simulink model "perfusion"  (Simulink 8.7)
settings: Solver=ode45  StartTime=0.0  StopTime=24  MaxStep=10  RelTol=1e-3
libraries: simulink x3
settings Model: Creator=asuri  LastModifiedBy=chnam  ExtModeAutoUpdateStatusClock=off
settings SolverCC: ZeroCrossControl=EnableAll
settings DataIOCC: SignalLoggingSaveFormat=ModelDataLogs  SaveOutput=off  SaveTime=off
settings OptimizationCC: BooleanDataType=off  ExpressionDepthLimit=2147483647  InitFltsAndDblsToZero=on
settings DebuggingCC: AlgebraicLoopMsg=error  SaveWithParameterizedLinksMsg=none  SignalResolutionControl=TryResolveAllWithWarning  MultiTaskDSMMsg=warning  MultiTaskCondExecSysMsg=none  InvalidFcnCallConnMsg=warning  FcnCallInpInsideContextMsg=UseLocalSettings  StateNameClashWarn=warning  StrictBusMsg=None
settings SFSimCC: SimParseCustomCode=off
settings GRTTargetCC: TargetFcnLib=ansi_tfl_tmw.mat  GeneratePreprocessorConditionals=Use local settings  CombineOutputUpdateFcns=off  GRTInterface=on

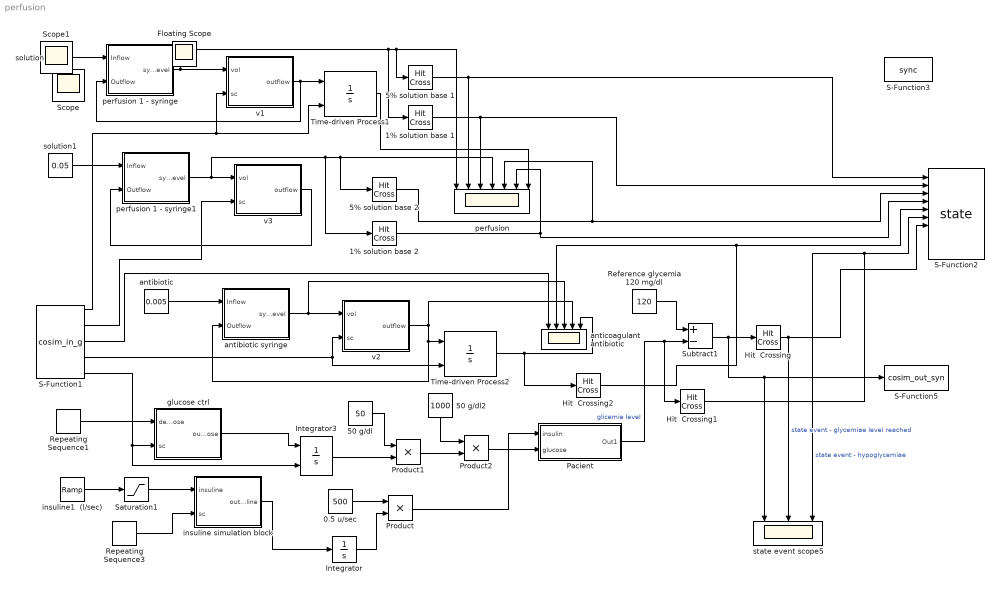
== system perfusion ==
  "0.5 u/sec " : Constant  Value=500
  1% solution base 1 : HitCross  HitCrossingOffset=0.075  HitCrossingDirection=falling  ZeroCross=off
  1% solution base 2 : HitCross  HitCrossingOffset=0.075  HitCrossingDirection=falling  ZeroCross=off
  5% solution base 1 : HitCross  HitCrossingOffset=0.1  HitCrossingDirection=falling  ZeroCross=off
  5% solution base 2 : HitCross  HitCrossingOffset=0.1  HitCrossingDirection=falling  ZeroCross=off
  50 g/dl : Constant  Value=50
  50 g/dl2 : Constant  Value=1000
  Hit  Crossing : HitCross
  Hit  Crossing1 : HitCross  HitCrossingOffset=60  HitCrossingDirection=falling  ZeroCross=off
  Hit  Crossing2 : HitCross  HitCrossingOffset=0.2  HitCrossingDirection=rising  ZeroCross=off
  Integrator : Integrator
  Integrator3 : Integrator  ExternalReset=either
  Pacient : Subsystem
  Product : Product  RndMeth=Zero
  Product1 : Product  RndMeth=Zero
  Product2 : Product  RndMeth=Zero
  "Reference glycemia 120 mg/dl " : Constant  Value=120
  Repeating Sequence1 : simulink/Sources/Repeating Sequence  rep_seq_t=[0 1]  rep_seq_y=[0 0.001]
  Repeating Sequence3 : simulink/Sources/Repeating Sequence  rep_seq_t=[0 1 2 3 4 5 6 7 8 9 10 11 12 13 14 15 16 17 18 19 20 21 22 23]  rep_seq_y=[0 0 0 0 0 0 0 0 0 0 0 0 0 0 0 0 0 0 0 1 0 0 0 0]
  S-Function1 : S-Function  Priority=0  FunctionName=cosim_in_g  Parameters=NpIn  SFunctionDeploymentMode=off  EnableBusSupport=off  mask{NpIn=5}
      mask prompts: NpIn "Number of input ports :"
      mask help: Simulink input ports number.
  S-Function2 : S-Function  FunctionName=state  Parameters=NS  SFunctionDeploymentMode=off  EnableBusSupport=off  mask{NS=10}
      mask prompts: NS "Number Of Input state events"
      mask help: Specify the number of input state events. It must be less than 10
  S-Function3 : S-Function  FunctionName=sync  SFunctionDeploymentMode=off  EnableBusSupport=off
  S-Function5 : S-Function  Priority=16  FunctionName=cosim_out_syn  Parameters=NoutPort  SFunctionDeploymentMode=off  EnableBusSupport=off  mask{NoutPort=1}
      mask prompts: NoutPort "Number of output ports :"
      mask help: 1. Simulink output ports number.
  Saturation1 : Saturate  UpperLimit=0.500  LowerLimit=1e-5
  Subtract1 : Sum  Inputs=+-
  Time-driven Process1 : Integrator  ExternalReset=either
  Time-driven Process2 : Integrator  ExternalReset=either
  antibiotic : Constant  Value=0.005
  antibiotic syringe : Subsystem
  anticoagulant antibiotic : Scope  NumInputPorts=5
  glucose ctrl : Subsystem
  insuline simulation block : Subsystem
  insuline1  (l/sec) : simulink/Sources/Ramp  slope=1e-4/3600  start=0  X0=0
  perfusion : Scope  NumInputPorts=7
  perfusion 1 - syringe : Subsystem
  perfusion 1 - syringe1 : Subsystem
  solution : Constant  Value=0.05
  solution1 : Constant  Value=0.05
  state event scope5 : Scope  NumInputPorts=3
  v1 : Subsystem
  v2 : Subsystem
  v3 : Subsystem
  Floating Scope : Scope
  Scope : Scope
  Scope1 : Scope
  wires:
  Repeating Sequence1/1 -> glucose ctrl/1(debit glucose)
  50 g/dl/1 -> Product1/1
  Integrator3/1 -> Product1/2
  glucose ctrl/1(outflow glucose) -> Integrator3/1
  Subtract1/1 -> Hit  Crossing/1, S-Function5/1, state event scope5/1
  "Reference glycemia 120 mg/dl "/1 -> Subtract1/1
  Pacient/1(Out1) -> Subtract1/2, Hit  Crossing1/1  "glicemie level"
  Product2/1 -> Pacient/2(glucose)
  Product1/1 -> Product2/2
  1% solution base 1/1 -> S-Function2/2, perfusion/3
  5% solution base 2/1 -> S-Function2/3, perfusion/5
  1% solution base 2/1 -> S-Function2/4, perfusion/6
  Hit  Crossing/1 -> S-Function2/7, state event scope5/2  "state event - glycemiae level reached"
  Hit  Crossing1/1 -> state event scope5/3, S-Function2/6  "state event - hypoglycemiae"
  S-Function1/3 -> anticoagulant antibiotic/1
  S-Function1/5 -> Integrator3/2, glucose ctrl/2(sc)
  5% solution base 1/1 -> perfusion/2, S-Function2/1
  50 g/dl2/1 -> Product2/1
  insuline1  (l/sec)/1 -> Saturation1/1
  Saturation1/1 -> insuline simulation block/1(insuline)
  insuline simulation block/1(outflow insuline) -> Integrator/1
  "0.5 u/sec "/1 -> Product/1
  Integrator/1 -> Product/2
  Product/1 -> Pacient/1(insulin)
  Repeating Sequence3/1 -> insuline simulation block/2(sc)
  antibiotic syringe/1(syringe level) -> v2/1(vol), anticoagulant antibiotic/3
  v2/1(outflow) -> antibiotic syringe/2(Outflow), Time-driven Process2/1, anticoagulant antibiotic/4
  Hit  Crossing2/1 -> S-Function2/5, anticoagulant antibiotic/2
  antibiotic/1 -> antibiotic syringe/1(Inflow)
  v1/1(outflow) -> Time-driven Process1/1, perfusion 1 - syringe/2(Outflow)
  perfusion 1 - syringe/1(syringe level) -> v1/1(vol), perfusion/1, 5% solution base 1/1, 1% solution base 1/1
  solution/1 -> perfusion 1 - syringe/1(Inflow)
  Time-driven Process1/1 -> perfusion/7
  S-Function1/1 -> v1/2(sc), Time-driven Process1/2
  Time-driven Process2/1 -> anticoagulant antibiotic/5, Hit  Crossing2/1
  S-Function1/4 -> v2/2(sc), Time-driven Process2/2
  solution1/1 -> perfusion 1 - syringe1/1(Inflow)
  v3/1(outflow) -> perfusion 1 - syringe1/2(Outflow)
  S-Function1/2 -> v3/2(sc)
  perfusion 1 - syringe1/1(syringe level) -> 1% solution base 2/1, 5% solution base 2/1, perfusion/4, v3/1(vol)

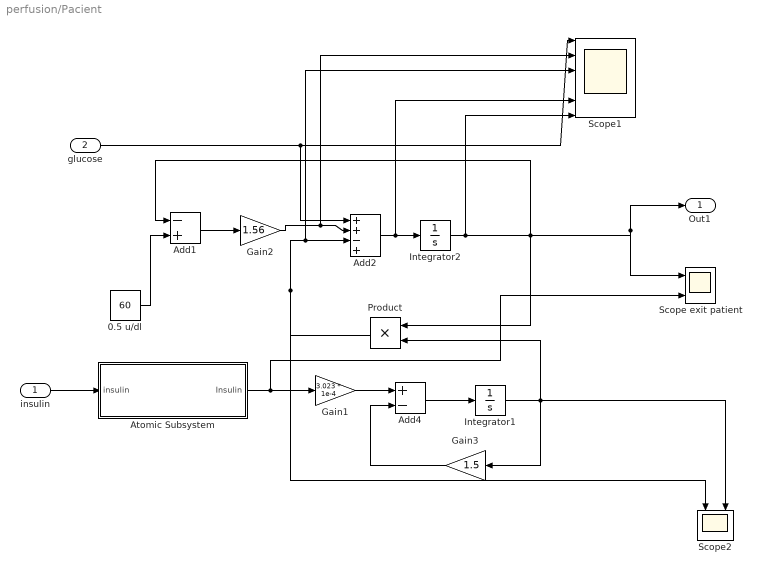
== system perfusion/Pacient ==
  insulin : Inport
  glucose : Inport  Port=2
  "0.5 u/dl " : Constant  Value=60
  Add1 : Sum  Inputs=-+
  Add2 : Sum  Inputs=++-+
  Add4 : Sum  Inputs=+-
  Atomic Subsystem : Subsystem  TreatAsAtomicUnit=on
  Gain1 : Gain  Gain=3.023 * 1e-4
  Gain2 : Gain  Gain=1.56
  Gain3 : Gain  Gain=1.5
  Integrator1 : Integrator
  Integrator2 : Integrator  InitialCondition=270
  Product : Product  RndMeth=Zero
  Scope exit patient : Scope  NumInputPorts=2
  Scope1 : Scope  NumInputPorts=6
  Scope2 : Scope  NumInputPorts=2
  Out1 : Outport
  wires:
  Add1/1 -> Gain2/1
  Add2/1 -> Integrator2/1, Scope1/5
  Integrator2/1 -> Add1/1, Product/1, Out1/1, Scope exit patient/1, Scope1/6
  Product/1 -> Scope2/1, Add2/3, Scope1/3
  Gain1/1 -> Add4/1
  Add4/1 -> Integrator1/1
  Integrator1/1 -> Gain3/1, Scope2/2, Product/2
  Gain3/1 -> Add4/2
  glucose/1 -> Add2/1, Scope1/1
  insulin/1 -> Atomic Subsystem/1(insulin)
  Atomic Subsystem/1(Insulin) -> Gain1/1, Scope exit patient/2
  Gain2/1 -> Add2/2, Scope1/2
  "0.5 u/dl "/1 -> Add1/2

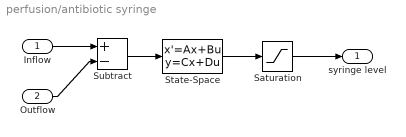
== system perfusion/antibiotic syringe ==
  Inflow : Inport
  Outflow : Inport  Port=2
  Saturation : Saturate  UpperLimit=100  LowerLimit=0
  State-Space : StateSpace  A=0  B=0.5  C=0.5  D=0  X0=3
  Subtract : Sum  Inputs=+-
  syringe level : Outport
  wires:
  Subtract/1 -> State-Space/1
  State-Space/1 -> Saturation/1
  Inflow/1 -> Subtract/1
  Saturation/1 -> syringe level/1
  Outflow/1 -> Subtract/2

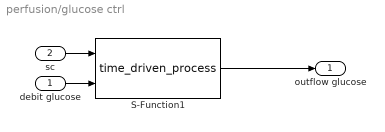
== system perfusion/glucose ctrl ==
  debit glucose : Inport
  sc : Inport  Port=2
  S-Function1 : S-Function  FunctionName=time_driven_process  Parameters=debitMax, debitMin  SFunctionDeploymentMode=off  EnableBusSupport=off  mask{debitMax=500, debitMin=0}
      mask prompts: debitMax "OutFlowMax"; debitMin "OutFlowMin"
  outflow glucose : Outport
  wires:
  S-Function1/1 -> outflow glucose/1
  sc/1 -> S-Function1/1
  debit glucose/1 -> S-Function1/2

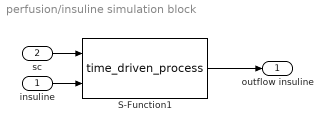
== system perfusion/insuline simulation block ==
  insuline : Inport
  sc : Inport  Port=2
  S-Function1 : S-Function  FunctionName=time_driven_process  Parameters=debitMax, debitMin  SFunctionDeploymentMode=off  EnableBusSupport=off  mask{debitMax=0.5, debitMin=0}
      mask prompts: debitMax "OutFlowMax"; debitMin "OutFlowMin"
  outflow insuline : Outport
  wires:
  S-Function1/1 -> outflow insuline/1
  sc/1 -> S-Function1/1
  insuline/1 -> S-Function1/2

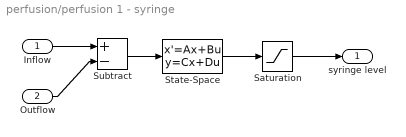
== system perfusion/perfusion 1 - syringe ==
  Inflow : Inport
  Outflow : Inport  Port=2
  Saturation : Saturate  UpperLimit=100  LowerLimit=0
  State-Space : StateSpace  A=0  B=0.5  C=0.5  D=0  X0=3
  Subtract : Sum  Inputs=+-
  syringe level : Outport
  wires:
  Subtract/1 -> State-Space/1
  State-Space/1 -> Saturation/1
  Inflow/1 -> Subtract/1
  Saturation/1 -> syringe level/1
  Outflow/1 -> Subtract/2

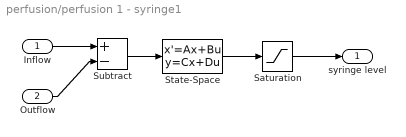
== system perfusion/perfusion 1 - syringe1 ==
  Inflow : Inport
  Outflow : Inport  Port=2
  Saturation : Saturate  UpperLimit=100  LowerLimit=0
  State-Space : StateSpace  A=0  B=0.5  C=0.5  D=0  X0=3
  Subtract : Sum  Inputs=+-
  syringe level : Outport
  wires:
  Subtract/1 -> State-Space/1
  State-Space/1 -> Saturation/1
  Inflow/1 -> Subtract/1
  Saturation/1 -> syringe level/1
  Outflow/1 -> Subtract/2

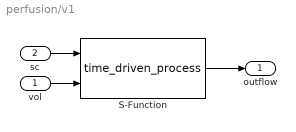
== system perfusion/v1 ==
  vol : Inport
  sc : Inport  Port=2
  S-Function : S-Function  FunctionName=time_driven_process  Parameters=debitMax, debitMin  SFunctionDeploymentMode=off  EnableBusSupport=off  mask{debitMax=0.003, debitMin=0.003}
      mask prompts: debitMax "OutFlowMax"; debitMin "OutFlowMin"
  outflow : Outport
  wires:
  S-Function/1 -> outflow/1
  sc/1 -> S-Function/1
  vol/1 -> S-Function/2

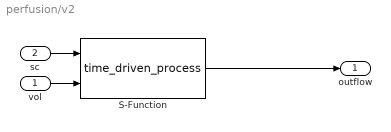
== system perfusion/v2 ==
  vol : Inport
  sc : Inport  Port=2
  S-Function : S-Function  FunctionName=time_driven_process  Parameters=debitMax, debitMin  SFunctionDeploymentMode=off  EnableBusSupport=off  mask{debitMax=0.003, debitMin=0.003}
      mask prompts: debitMax "OutFlowMax"; debitMin "OutFlowMin"
  outflow : Outport
  wires:
  sc/1 -> S-Function/1
  vol/1 -> S-Function/2
  S-Function/1 -> outflow/1

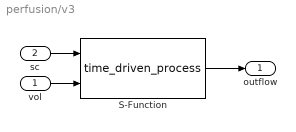
== system perfusion/v3 ==
  vol : Inport
  sc : Inport  Port=2
  S-Function : S-Function  FunctionName=time_driven_process  Parameters=debitMax, debitMin  SFunctionDeploymentMode=off  EnableBusSupport=off  mask{debitMax=0.003, debitMin=0.003}
      mask prompts: debitMax "OutFlowMax"; debitMin "OutFlowMin"
  outflow : Outport
  wires:
  S-Function/1 -> outflow/1
  sc/1 -> S-Function/1
  vol/1 -> S-Function/2

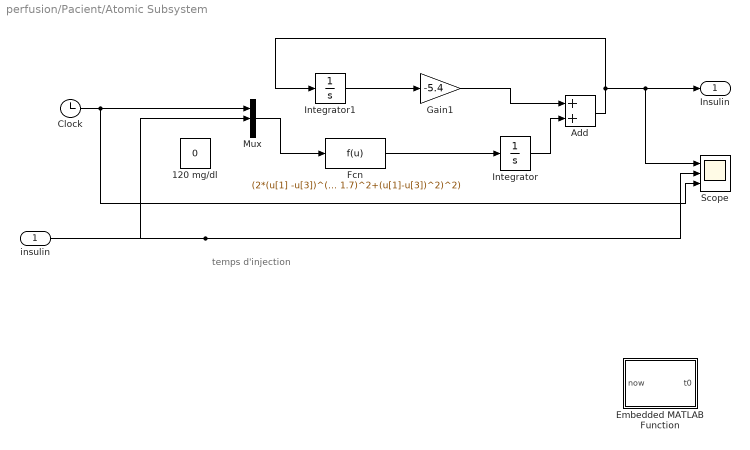
== system perfusion/Pacient/Atomic Subsystem ==
  note: temps d'injection
  insulin : Inport
  120 mg/dl : Constant  Value=0
  Add : Sum
  Clock : Clock
  Embedded MATLAB Function : MATLAB Function  TreatAsAtomicUnit=on
  Fcn : Fcn  Expr=(2*(u[1] -u[3])^(2-1)*u[2] * (0.05*u[2] + 1.7)^2)/(120*( (0.05*u[2] + 1.7)^2+(u[1]-u[3])^2)^2)
  Gain1 : Gain  Gain=-5.4
  Integrator : Integrator
  Integrator1 : Integrator
  Mux : Mux  Inputs=3
  Scope : Scope  NumInputPorts=3
  Insulin : Outport
  wires:
  Fcn/1 -> Integrator/1
  Integrator/1 -> Add/2
  Gain1/1 -> Add/1
  Add/1 -> Scope/1, Insulin/1, Integrator1/1
  insulin/1 -> Mux/2, Scope/2
  Mux/1 -> Fcn/1
  Clock/1 -> Mux/1, Scope/3
  Integrator1/1 -> Gain1/1

== matlab function Pacient/Atomic Subsystem/Embedded MATLAB Function ==
  data: now input double; t0 output double
function t0 = fcn(now)
% This block supports an embeddable subset of the MATLAB language.
% See the help menu for details. 

if now < 3600*1
    t0 = 0;
else
    t0 = 3600*1;
end
